simulink subsystem "wheel_encoder"  (R2022b)
settings: Solver=VariableStepAuto  StartTime=0.0  StopTime=10.0  RelTol=1e-3
model mask{variant=Sampling, R=95, n=24, invert=off, PinA=D5, PinB=D6}
  mask prompts: variant "Implementation"; R "Wheel Radius [mm]"; n "Pulses Per Rotation"; invert "Reverse Direction"; PinA "Pin A"; PinB "Pin B"
undefined symbols (not defined in the file): t_step
libraries: mbedblockslib x8, eeQuadratureDecoder x1
settings Model: Creator=micha  LastModifiedBy=micha

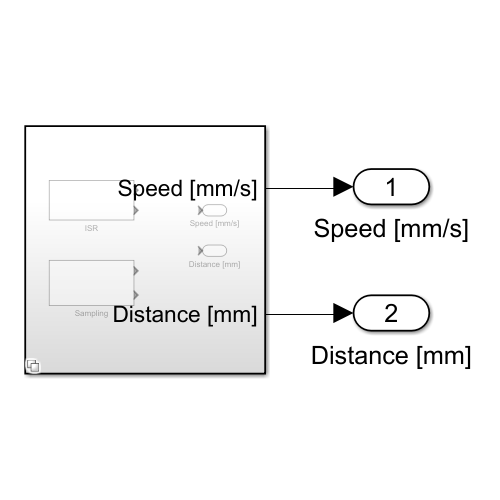
[thumbnail: Simulink's stored preview of the top-level diagram]
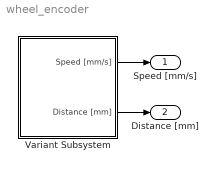
== system wheel_encoder ==
  Variant Subsystem : Subsystem  Variant=on
  Speed [mm/s] : Outport
  Distance [mm] : Outport  Port=2
  wires:
  Variant Subsystem/2(Distance [mm]) -> Distance [mm]/1
  Variant Subsystem/1(Speed [mm/s]) -> Speed [mm/s]/1

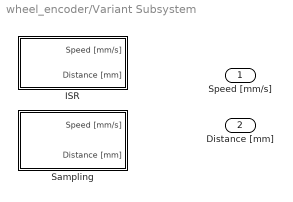
== system wheel_encoder/Variant Subsystem ==
  ISR : Subsystem  VariantControl=variant == 1
  Sampling : Subsystem  VariantControl=variant == 2
  Speed [mm/s] : Outport
  Distance [mm] : Outport  Port=2

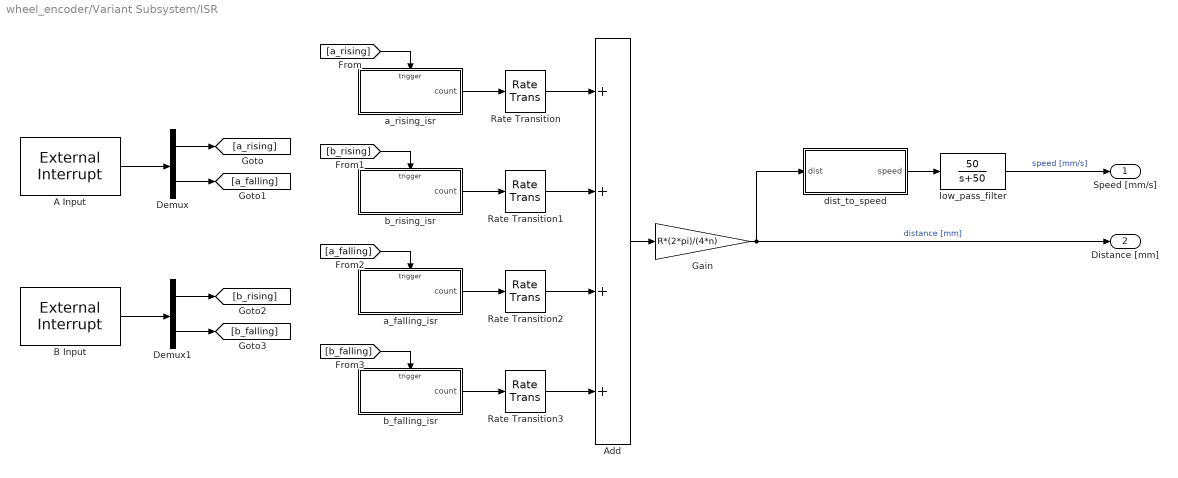
== system wheel_encoder/Variant Subsystem/ISR ==
  A Input : mbedblockslib/External Interrupt  Pin=D2  Mode=No pull-up or pull-down  EdgeSelection=Either  VectorFcnCallOutput=on  SimulationInput=off  InitialPinStatus=false  BlockPlatform=nucleo
      settings: LibrarySourceBlock=stmnucleorootlib/Common/External Interrupt
  Add : Sum  Inputs=++++
  B Input : mbedblockslib/External Interrupt  Pin=D3  Mode=No pull-up or pull-down  EdgeSelection=Either  VectorFcnCallOutput=on  SimulationInput=off  InitialPinStatus=false  BlockPlatform=nucleo
      settings: LibrarySourceBlock=stmnucleorootlib/Common/External Interrupt
  Demux : Demux  Outputs=2
  Demux1 : Demux  Outputs=2
  Gain : Gain  Gain=R*(2*pi)/(4*n)
  Rate Transition{,1..3} (4 alike) : RateTransition  Deterministic=off
  a_falling_isr : Subsystem  TreatAsAtomicUnit=on
  a_rising_isr : Subsystem  TreatAsAtomicUnit=on
  b_falling_isr : Subsystem  TreatAsAtomicUnit=on
  b_rising_isr : Subsystem  TreatAsAtomicUnit=on
  dist_to_speed : Subsystem
  low_pass_filter : TransferFcn  Numerator=[50]  Denominator=[1 50]
  Speed [mm/s] : Outport
  Distance [mm] : Outport  Port=2
  wires:
  dist_to_speed/1(speed) -> low_pass_filter/1
  Rate Transition3/1 -> Add/4
  Rate Transition2/1 -> Add/3
  [b_falling] -> b_falling_isr/Trigger
  [a_falling] -> a_falling_isr/Trigger
  [b_rising] -> b_rising_isr/Trigger
  [a_rising] -> a_rising_isr/Trigger
  a_falling_isr/1(count) -> Rate Transition2/1
  b_falling_isr/1(count) -> Rate Transition3/1
  Demux1/1 -> [b_rising]
  B Input/1 -> Demux1/1
  Demux1/2 -> [b_falling]
  Demux/2 -> [a_falling]
  Demux/1 -> [a_rising]
  Rate Transition1/1 -> Add/2
  Gain/1 -> dist_to_speed/1(dist), Distance [mm]/1  "distance [mm]"
  A Input/1 -> Demux/1
  b_rising_isr/1(count) -> Rate Transition1/1
  Add/1 -> Gain/1
  a_rising_isr/1(count) -> Rate Transition/1
  low_pass_filter/1 -> Speed [mm/s]/1  "speed [mm/s]"
  Rate Transition/1 -> Add/1

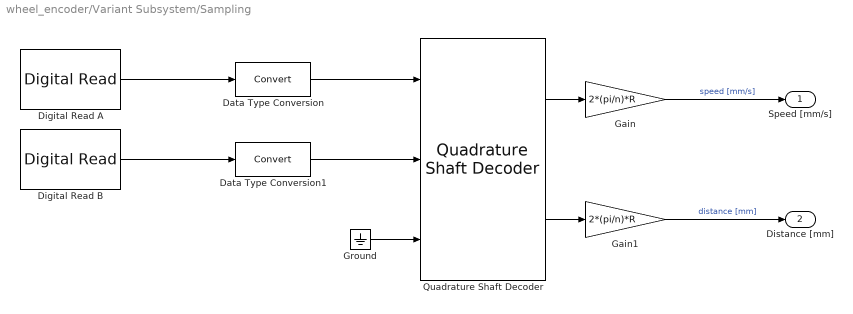
== system wheel_encoder/Variant Subsystem/Sampling ==
  Data Type Conversion : DataTypeConversion  SaturateOnIntegerOverflow=off  RndMeth=Floor
  Data Type Conversion1 : DataTypeConversion  SaturateOnIntegerOverflow=off  RndMeth=Floor
  Digital Read A : mbedblockslib/Digital Read  Pin=D2  Direction=input  SampleTime=t_step
      settings: LibrarySourceBlock=stmnucleorootlib/Common/Digital Read
  Digital Read B : mbedblockslib/Digital Read  Pin=D3  Direction=input  SampleTime=t_step
      settings: LibrarySourceBlock=stmnucleorootlib/Common/Digital Read
  Gain : Gain  Gain=2*(pi/n)*R
  Gain1 : Gain  Gain=2*(pi/n)*R
  Ground : Ground
  Quadrature Shaft Decoder : eeQuadratureDecoder/Quadrature Shaft Decoder  NPulse=n  Ts=t_step
      settings: LibrarySourceBlock=|
      | ee_sl_lib/Observers/Quadrature Shaft
      | Decoder
  Speed [mm/s] : Outport
  Distance [mm] : Outport  Port=2
  wires:
  Quadrature Shaft Decoder/2 -> Gain1/1
  Gain1/1 -> Distance [mm]/1  "distance [mm]"
  Quadrature Shaft Decoder/1 -> Gain/1
  Gain/1 -> Speed [mm/s]/1  "speed [mm/s]"
  Ground/1 -> Quadrature Shaft Decoder/3
  Digital Read B/1 -> Data Type Conversion1/1
  Digital Read A/1 -> Data Type Conversion/1
  Data Type Conversion/1 -> Quadrature Shaft Decoder/1
  Data Type Conversion1/1 -> Quadrature Shaft Decoder/2

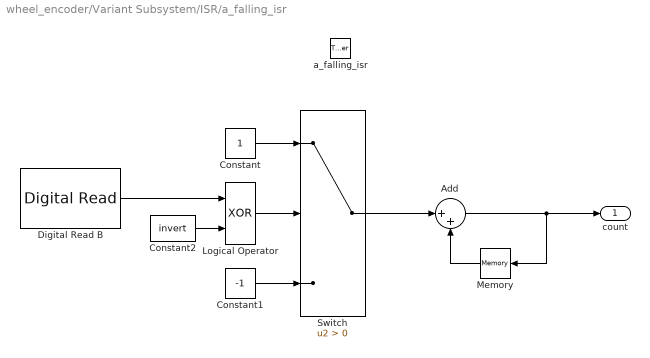
== system wheel_encoder/Variant Subsystem/ISR/a_falling_isr ==
  a_falling_isr : TriggerPort  TriggerType=function-call  VariantControl=(inherit)
  Add : Sum  Inputs=|++
  Constant : Constant
  Constant1 : Constant  Value=-1
  Constant2 : Constant  Value=invert
  Digital Read B : mbedblockslib/Digital Read  Pin=D3  Direction=input  SampleTime=-1
      settings: LibrarySourceBlock=stmnucleorootlib/Common/Digital Read
  Logical Operator : Logic  Operator=XOR  AllPortsSameDT=off  OutDataTypeStr=boolean
  Memory : Memory  InheritSampleTime=on
  Switch : Switch  Criteria=u2 > Threshold  SaturateOnIntegerOverflow=off  InputSameDT=off
  count : Outport
  wires:
  Switch/1 -> Add/1
  Digital Read B/1 -> Logical Operator/1
  Constant1/1 -> Switch/3
  Add/1 -> Memory/1, count/1
  Memory/1 -> Add/2
  Constant2/1 -> Logical Operator/2
  Logical Operator/1 -> Switch/2
  Constant/1 -> Switch/1

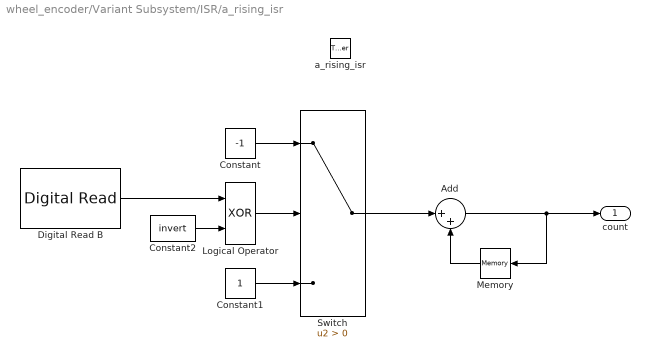
== system wheel_encoder/Variant Subsystem/ISR/a_rising_isr ==
  a_rising_isr : TriggerPort  TriggerType=function-call  VariantControl=(inherit)
  Add : Sum  Inputs=|++
  Constant : Constant  Value=-1
  Constant1 : Constant
  Constant2 : Constant  Value=invert
  Digital Read B : mbedblockslib/Digital Read  Pin=D3  Direction=input  SampleTime=-1
      settings: LibrarySourceBlock=stmnucleorootlib/Common/Digital Read
  Logical Operator : Logic  Operator=XOR  AllPortsSameDT=off  OutDataTypeStr=boolean
  Memory : Memory  InheritSampleTime=on
  Switch : Switch  Criteria=u2 > Threshold  SaturateOnIntegerOverflow=off  InputSameDT=off
  count : Outport
  wires:
  Switch/1 -> Add/1
  Digital Read B/1 -> Logical Operator/1
  Constant1/1 -> Switch/3
  Add/1 -> Memory/1, count/1
  Memory/1 -> Add/2
  Constant2/1 -> Logical Operator/2
  Logical Operator/1 -> Switch/2
  Constant/1 -> Switch/1

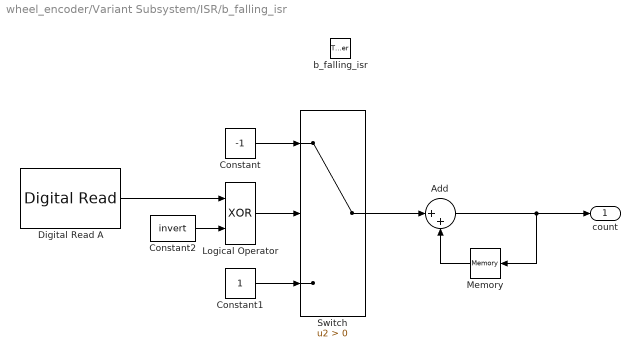
== system wheel_encoder/Variant Subsystem/ISR/b_falling_isr ==
  b_falling_isr : TriggerPort  TriggerType=function-call  VariantControl=(inherit)
  Add : Sum  Inputs=|++
  Constant : Constant  Value=-1
  Constant1 : Constant
  Constant2 : Constant  Value=invert
  Digital Read A : mbedblockslib/Digital Read  Pin=D2  Direction=input  SampleTime=-1
      settings: LibrarySourceBlock=stmnucleorootlib/Common/Digital Read
  Logical Operator : Logic  Operator=XOR  AllPortsSameDT=off  OutDataTypeStr=boolean
  Memory : Memory  InheritSampleTime=on
  Switch : Switch  Criteria=u2 > Threshold  SaturateOnIntegerOverflow=off  InputSameDT=off
  count : Outport
  wires:
  Switch/1 -> Add/1
  Digital Read A/1 -> Logical Operator/1
  Constant1/1 -> Switch/3
  Add/1 -> Memory/1, count/1
  Memory/1 -> Add/2
  Constant2/1 -> Logical Operator/2
  Logical Operator/1 -> Switch/2
  Constant/1 -> Switch/1

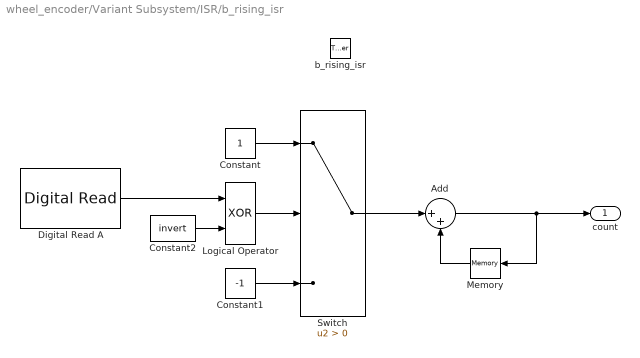
== system wheel_encoder/Variant Subsystem/ISR/b_rising_isr ==
  b_rising_isr : TriggerPort  TriggerType=function-call  VariantControl=(inherit)
  Add : Sum  Inputs=|++
  Constant : Constant
  Constant1 : Constant  Value=-1
  Constant2 : Constant  Value=invert
  Digital Read A : mbedblockslib/Digital Read  Pin=D2  Direction=input  SampleTime=-1
      settings: LibrarySourceBlock=stmnucleorootlib/Common/Digital Read
  Logical Operator : Logic  Operator=XOR  AllPortsSameDT=off  OutDataTypeStr=boolean
  Memory : Memory  InheritSampleTime=on
  Switch : Switch  Criteria=u2 > Threshold  SaturateOnIntegerOverflow=off  InputSameDT=off
  count : Outport
  wires:
  Switch/1 -> Add/1
  Digital Read A/1 -> Logical Operator/1
  Constant1/1 -> Switch/3
  Add/1 -> Memory/1, count/1
  Memory/1 -> Add/2
  Constant2/1 -> Logical Operator/2
  Logical Operator/1 -> Switch/2
  Constant/1 -> Switch/1

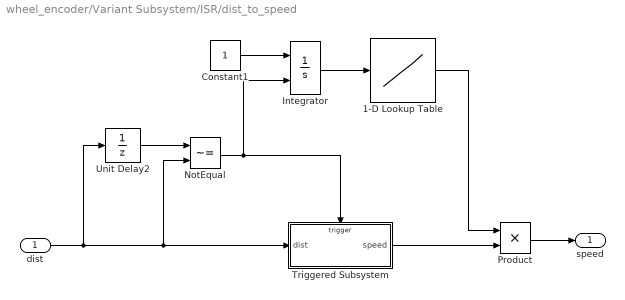
== system wheel_encoder/Variant Subsystem/ISR/dist_to_speed ==
  dist : Inport
  1-D Lookup Table : Lookup_n-D  NumberOfTableDimensions=1  BreakpointsForDimension1=[0, 0.25, 0.5]  Table=[1, 1, 0]  ExtrapMethod=Clip  UseLastTableValue=on  InternalRulePriority=Speed  RndMeth=Simplest
  Constant1 : Constant
  Integrator : Integrator  ExternalReset=rising
  NotEqual : RelationalOperator  Operator=~=  OutDataTypeStr=boolean  RndMeth=Simplest  InputSameDT=off
  Product : Product
  Triggered Subsystem : Subsystem  TreatAsAtomicUnit=on
  Unit Delay2 : UnitDelay  SampleTime=-1  HasFrameUpgradeWarning=on
  speed : Outport
  wires:
  Unit Delay2/1 -> NotEqual/1
  dist/1 -> NotEqual/2, Triggered Subsystem/1(dist), Unit Delay2/1
  Product/1 -> speed/1
  Triggered Subsystem/1(speed) -> Product/2
  Constant1/1 -> Integrator/1
  NotEqual/1 -> Triggered Subsystem/Trigger, Integrator/2
  1-D Lookup Table/1 -> Product/1
  Integrator/1 -> 1-D Lookup Table/1

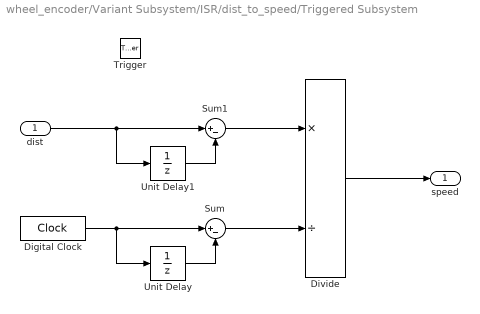
== system wheel_encoder/Variant Subsystem/ISR/dist_to_speed/Triggered Subsystem ==
  dist : Inport
  Trigger : TriggerPort  VariantControl=(inherit)
  Digital Clock : DigitalClock  SampleTime=-1
  Divide : Product  Inputs=*/
  Sum : Sum  Inputs=|+-
  Sum1 : Sum  Inputs=|+-
  Unit Delay : UnitDelay  SampleTime=-1  HasFrameUpgradeWarning=on
  Unit Delay1 : UnitDelay  SampleTime=-1  HasFrameUpgradeWarning=on
  speed : Outport
  wires:
  Divide/1 -> speed/1
  Sum/1 -> Divide/2
  Sum1/1 -> Divide/1
  dist/1 -> Sum1/1, Unit Delay1/1
  Unit Delay1/1 -> Sum1/2
  Unit Delay/1 -> Sum/2
  Digital Clock/1 -> Sum/1, Unit Delay/1
